simulink model "model_graphicSim"  (R2022a)
settings: Solver=FixedStepAuto  StartTime=0.0  StopTime=inf  RelTol=1e-3
values from neighbouring files (symbols this model uses):
  A = 9    [A_circuit_V2_25000.mat]    (also in A_circuit_V2_3167.mat; A_circuit_V3_30000.mat; A_circuit_V3_60000.mat; Configuration.m)
  d = 699840    [A_circuit_V2_25000.mat]    (also in A_circuit_V2_3167.mat; A_circuit_V3_30000.mat; A_circuit_V3_60000.mat; Configuration.m)
  egoID = 1    [A_circuit_V2_25000.mat]    (also in A_circuit_V2_3167.mat; A_circuit_V3_30000.mat; A_circuit_V3_60000.mat; Configuration.m)
  frontDistCG = 3.7    [A_circuit_V2_25000.mat]    (also in A_circuit_V2_3167.mat; A_circuit_V3_30000.mat; A_circuit_V3_60000.mat; Configuration.m)
  gridvx = [-5 -4.72222222222 -4.44444444444 -4.16666666667 -3.88888888889 -3.61111111111 -3.33333333333 -3.05555555556 -2.77777777778 -2.5 0 0.277777777778 ... (70 elements, 10x7)]    [A_circuit_V2_25000.mat]    (also in A_circuit_V2_3167.mat; A_circuit_V3_30000.mat; A_circuit_V3_60000.mat; circuit_10000_P2.mat)
  gridvy = [-70 -68.4444444444 -66.8888888889 -65.3333333333 -63.7777777778 -62.2222222222 -60.6666666667 -59.1111111111 -57.5555555556 -56 -50 -48.4444444444 ... (70 elements, 10x7)]    [A_circuit_V2_25000.mat]    (also in A_circuit_V2_3167.mat; A_circuit_V3_30000.mat; A_circuit_V3_60000.mat; circuit_10000_P2.mat)
  gridx = [-85 -84.6666666667 -84.3333333333 -84 -83.6666666667 -83.3333333333 -83 -82.6666666667 -82.3333333333 -82 -55 -54.6666666667 ... (70 elements, 10x7)]    [A_circuit_V2_25000.mat]    (also in A_circuit_V2_3167.mat; A_circuit_V3_30000.mat; A_circuit_V3_60000.mat; circuit_10000_P2.mat)
  gridy = [-70 -69.3333333333 -68.6666666667 -68 -67.3333333333 -66.6666666667 -66 -65.3333333333 -64.6666666667 -64 -50 -49.3333333333 ... (70 elements, 10x7)]    [A_circuit_V2_25000.mat]    (also in A_circuit_V2_3167.mat; A_circuit_V3_30000.mat; A_circuit_V3_60000.mat; circuit_10000_P2.mat)
  gridyaw = [-504 -489.6 -475.2 -460.8 -446.4 -432 -417.6 -403.2 -388.8 -374.4 -360 -345.6 ... (70 elements, 10x7)]    [A_circuit_V2_25000.mat]    (also in A_circuit_V2_3167.mat; A_circuit_V3_30000.mat; A_circuit_V3_60000.mat; circuit_10000_P2.mat)
  lb_angSt = -1080    [A_circuit_V2_25000.mat]    (also in A_circuit_V2_3167.mat; A_circuit_V3_30000.mat; A_circuit_V3_60000.mat; Configuration.m = -900)
  lbvx = 0    [A_circuit_V2_25000.mat]    (also in A_circuit_V2_3167.mat; A_circuit_V3_30000.mat; A_circuit_V3_60000.mat; Configuration.m = -2)
  lbvy = -50    [A_circuit_V2_25000.mat]    (also in A_circuit_V2_3167.mat; A_circuit_V3_30000.mat; A_circuit_V3_60000.mat; Configuration.m = -20)
  lbx = -55    [A_circuit_V2_25000.mat]    (also in A_circuit_V2_3167.mat; A_circuit_V3_30000.mat; A_circuit_V3_60000.mat; Configuration.m = 0)
  lby = -50    [A_circuit_V2_25000.mat]    (also in A_circuit_V2_3167.mat; A_circuit_V3_30000.mat; A_circuit_V3_60000.mat; Configuration.m = 2)
  lbyaw = -90    [Configuration.m]    (also in Configuration_circuit.m = -360; Configuration_circuit_V2.m = -360; Configuration_curve.m = -360; Configuration_curve_2.m = -360)
  leftDistCG = 0.9    [A_circuit_V2_25000.mat]    (also in A_circuit_V2_3167.mat; A_circuit_V3_30000.mat; A_circuit_V3_60000.mat; Configuration.m)
  M = 5    [A_circuit_V2_25000.mat]    (also in A_circuit_V2_3167.mat; A_circuit_V3_30000.mat; A_circuit_V3_60000.mat; Configuration.m)
  N = 10    [A_circuit_V2_25000.mat]    (also in A_circuit_V2_3167.mat; A_circuit_V3_30000.mat; A_circuit_V3_60000.mat; Configuration.m)
  passo_steerang = 45    [A_circuit_V2_25000.mat]    (also in A_circuit_V2_3167.mat; A_circuit_V3_30000.mat; A_circuit_V3_60000.mat; Configuration.m = 180)
  passo_v = 0.5    [A_circuit_V2_25000.mat]    (also in A_circuit_V2_3167.mat; A_circuit_V3_30000.mat; A_circuit_V3_60000.mat; Configuration.m)
  retroDistCG = 1    [A_circuit_V2_25000.mat]    (also in A_circuit_V2_3167.mat; A_circuit_V3_30000.mat; A_circuit_V3_60000.mat; Configuration.m)
  safetyDist = 0.5    [A_circuit_V2_25000.mat]    (also in A_circuit_V2_3167.mat; A_circuit_V3_30000.mat; A_circuit_V3_60000.mat; Configuration.m)
  Ts = 0.1    [A_circuit_V2_25000.mat]    (also in A_circuit_V2_3167.mat; A_circuit_V3_30000.mat; A_circuit_V3_60000.mat; Configuration.m)
  ub_angSt = 1080    [A_circuit_V2_25000.mat]    (also in A_circuit_V2_3167.mat; A_circuit_V3_30000.mat; A_circuit_V3_60000.mat; Configuration.m = 900)
  ubvx = 25    [A_circuit_V2_25000.mat]    (also in A_circuit_V2_3167.mat; A_circuit_V3_30000.mat; A_circuit_V3_60000.mat; Configuration.m = 2)
  ubvy = 50    [A_circuit_V2_25000.mat]    (also in A_circuit_V2_3167.mat; A_circuit_V3_30000.mat; A_circuit_V3_60000.mat; Configuration.m = 20)
  ubx = 95    [A_circuit_V2_25000.mat]    (also in A_circuit_V2_3167.mat; A_circuit_V3_30000.mat; A_circuit_V3_60000.mat; Configuration.m = 25)
  uby = 50    [A_circuit_V2_25000.mat]    (also in A_circuit_V2_3167.mat; A_circuit_V3_30000.mat; A_circuit_V3_60000.mat; Configuration.m = 10)
  ubyaw = 90    [Configuration.m]    (also in Configuration_circuit.m = 360; Configuration_circuit_V2.m = 360; Configuration_curve.m = 360; Configuration_curve_2.m = 360)
  w = [0 0 0 0 0 0 0 0 0 0 0 0 ... (699840 elements, 699840x1)]    [A_circuit_V2_25000.mat]    (also in A_circuit_V2_3167.mat; A_circuit_V3_30000.mat; A_circuit_V3_60000.mat; circuit_10000_P2.mat)
  x_0 = 2*rand+19    [Configuration.m]    (also in Configuration_circuit.m = -30; Configuration_circuit_V2.m = 0; Configuration_curve.m = 5; Configuration_curve_2.m = 5)
  y_0 = -(3.5*rand+2)    [Configuration.m]    (also in Configuration_circuit.m = -(-20 - rand*6); Configuration_circuit_V2.m = -(-29.5 - rand*7); Configuration_curve.m = -(1-2.1*rand); Configuration_curve_2.m = -(1-2.1*rand))
undefined symbols (not defined in the file or in its folder): deg, driving, rad, s
libraries: drivingscenarioandsensors x17, simulink_extras x2, sim3dlib x1, sim3dautolib x1, aerolibconvert2 x1, vehdynlibsteering x1, autolibshared x1
(part 1 of 6)
settings Model: Creator=User  LastModifiedBy=User

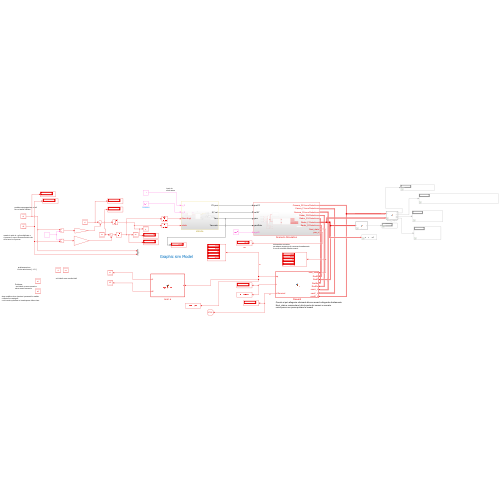
[thumbnail: Simulink's stored preview of the top-level diagram]
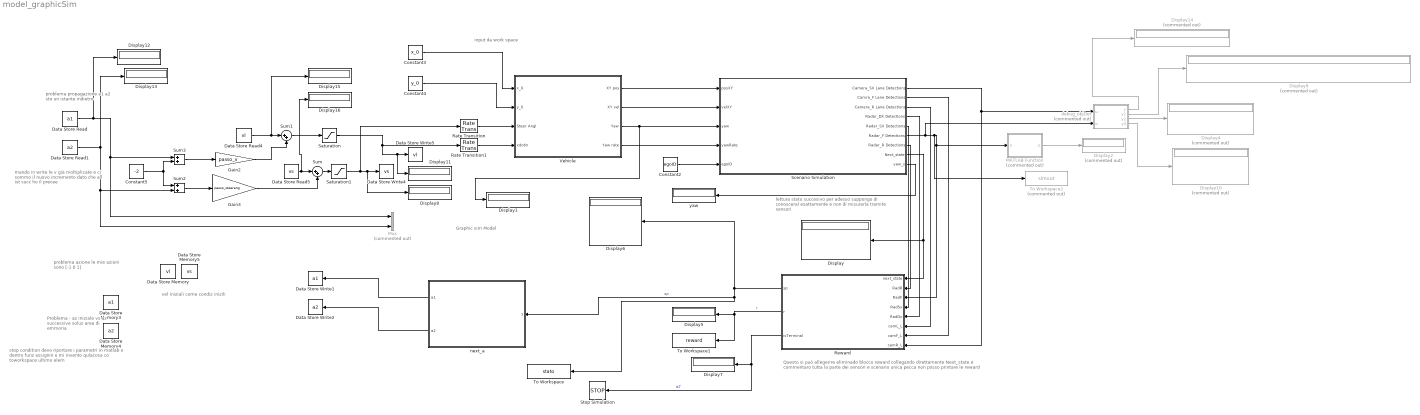
== system model_graphicSim ==
  note: Questo si può allegerire eliminado blocco reward collegando direttamente
      | Next_state e commentaro tutta la parte dei sensori e scenario
      | unica pecca non posso printare le reward
  note: mando in write le v già moltiplicate e
      | ci sommo il nuovo incremento dato che
      | all ist succ ho il precee
  note: problema azione
      | le mie azioni sono [-1 0 1]
  note: vel iniziali come condiz inizili
  note: stop condition devo riportare i parametri in matlab
      | o dentro funz assignin
      | o mi invento qulacosa co toworkspace ultimo elem
  note: Problema
      | - az iniziale vs az successive
      | soluz area di emmoria
  note: problema propagazione a1 a2
      | sto un istante indietro
  note: input da work space
  note: Graphic sim Model
  note: lettura stato succesivo
      | per adesso suppongo di conosceral esattamente
      | e non di misurarla tramite sensori
  Constant2 : Constant  Value=egoID
  Constant3 : Constant  Value=x_0
  Constant4 : Constant  Value=y_0
  Constant5 : Constant  Value=-2
  Data Store Memory : DataStoreMemory  DataStoreName=vl  WriteAfterWriteMsg=warning  ShowAdditionalParam=off
  Data Store Memory3 : DataStoreMemory  DataStoreName=a1  WriteAfterWriteMsg=warning  InitialValue=az_1  VectorParams1D=off  ShowAdditionalParam=off  OutDataTypeStr=double
  Data Store Memory4 : DataStoreMemory  DataStoreName=a2  WriteAfterWriteMsg=warning  InitialValue=az_2  VectorParams1D=off  ShowAdditionalParam=off  OutDataTypeStr=double
  Data Store Memory5 : DataStoreMemory  DataStoreName=vs  WriteAfterWriteMsg=warning  ShowAdditionalParam=off
  Data Store Read : DataStoreRead  DataStoreName=a1  IndexOptions=Index vector (dialog)  Indices=1  OutputSizes=1
  Data Store Read1 : DataStoreRead  DataStoreName=a2  IndexOptions=Index vector (dialog)  Indices=1  OutputSizes=1
  Data Store Read4 : DataStoreRead  DataStoreName=vl  IndexOptions=Index vector (dialog)  Indices=1  OutputSizes=1
  Data Store Read5 : DataStoreRead  DataStoreName=vs  IndexOptions=Index vector (dialog)  Indices=1  OutputSizes=1
  Data Store Write1 : DataStoreWrite  DataStoreName=a1  IndexOptions=Index vector (dialog)  Indices=1  OutputSizes=1
  Data Store Write2 : DataStoreWrite  DataStoreName=a2  IndexOptions=Index vector (dialog)  Indices=1  OutputSizes=1
  Data Store Write4 : DataStoreWrite  DataStoreName=vs  IndexOptions=Index vector (dialog)  Indices=1  OutputSizes=1
  Data Store Write5 : DataStoreWrite  DataStoreName=vl  IndexOptions=Index vector (dialog)  Indices=1  OutputSizes=1
  Display{,1,5..8,11..13,15..16} (11 alike) : Display
  Display{2,4,9..10,14} (5 alike) : Display  Commented=on
  Gain2 : Gain  Gain=passo_v
  Gain3 : Gain  Gain=passo_steerang
  MATLAB Function : MATLAB Function  Commented=on  TreatAsAtomicUnit=on
  Mux : Mux  Commented=on  Inputs=2
  Rate Transition : RateTransition
  Rate Transition1 : RateTransition
  Reward : MATLAB Function  TreatAsAtomicUnit=on
  Saturation : Saturate  UpperLimit=ubvx  LowerLimit=lbvx
  Saturation1 : Saturate  UpperLimit=ub_angSt  LowerLimit=lb_angSt
  Scenario Simulation : Subsystem
  Stop Simulation : Stop
  Sum : Sum  Inputs=|++
  Sum1 : Sum  Inputs=|++
  Sum2 : Sum
  Sum3 : Sum
  To Workspace : ToWorkspace  VariableName=stato  SampleTime=-1
  To Workspace1 : ToWorkspace  VariableName=reward  SampleTime=-1
  To Workspace2 : ToWorkspace  Commented=on  VariableName=simout  SaveFormat=Timeseries  SampleTime=-1
  Vehicle : Subsystem
  debug_objDet : MATLAB Function  Commented=on  TreatAsAtomicUnit=on
  next_a : MATLAB Function  TreatAsAtomicUnit=on
  yaw : Display
  wires:
  Saturation1/1 -> Rate Transition/1, Display8/1, Data Store Write4/1
  Rate Transition/1 -> Vehicle/3(Steer Angl)
  Reward/2(r) -> To Workspace1/1, Display5/1  "r"
  Vehicle/3(Yaw) -> Display1/1, Scenario Simulation/3(yaw)
  Gain2/1 -> Sum1/2
  Sum3/1 -> Gain2/1
  Data Store Read5/1 -> Display16/1, Sum/1
  Data Store Read/1 -> Display12/1, Sum3/1, Mux/1
  Sum1/1 -> Saturation/1
  Sum/1 -> Saturation1/1
  Sum2/1 -> Gain3/1
  Saturation/1 -> Data Store Write5/1, Display11/1, Rate Transition1/1
  Reward/3(isTerminal) -> Stop Simulation/1, Display7/1  "isT"
  Data Store Read1/1 -> Display13/1, Sum2/2, Mux/2
  Constant5/1 -> Sum3/2, Sum2/1
  Gain3/1 -> Sum/2
  Constant3/1 -> Vehicle/1(x_0)
  Data Store Read4/1 -> Display15/1, Sum1/1
  Reward/1(sp) -> Display6/1, To Workspace/1, next_a/1(s)  "sp"
  Vehicle/4(Yaw rate) -> Scenario Simulation/4(yawRate)
  Constant2/1 -> Scenario Simulation/5(egoID)
  Vehicle/2(XY vel) -> Scenario Simulation/2(velXY)
  Rate Transition1/1 -> Vehicle/4(xdotin)
  Vehicle/1(XY pos) -> Scenario Simulation/1(posXY)
  Constant4/1 -> Vehicle/2(y_0)
  next_a/1(a1) -> Data Store Write1/1
  next_a/2(a2) -> Data Store Write2/1
  Scenario Simulation/7(Radar_R Detections) -> Reward/2(RadR)
  Scenario Simulation/5(" Radar_SX Detections") -> Reward/4(RadSx)
  Scenario Simulation/4(Radar_DX Detections) -> Reward/5(RadDx)
  Scenario Simulation/3(Camera_R Lane Detections) -> Reward/6(camL_L)
  Scenario Simulation/2(" Camra_F Lane Detections") -> Reward/7(camF_L)
  Scenario Simulation/1(Camera_SX Lane Detections) -> debug_objDet/1(u), Reward/8(camR_L)
  Scenario Simulation/8(Next_state) -> Display/1, Reward/1(next_state)
  Scenario Simulation/9(yaw_s) -> yaw/1
  Scenario Simulation/6(Radar_F Detections) -> debug_objDet/2(o), MATLAB Function/1(u), Reward/3(RadF), To Workspace2/1
  MATLAB Function/1(y) -> Display2/1
  debug_objDet/4(y3) -> Display10/1
  debug_objDet/1(y) -> Display14/1
  debug_objDet/3(y2) -> Display4/1
  debug_objDet/2(y1) -> Display9/1

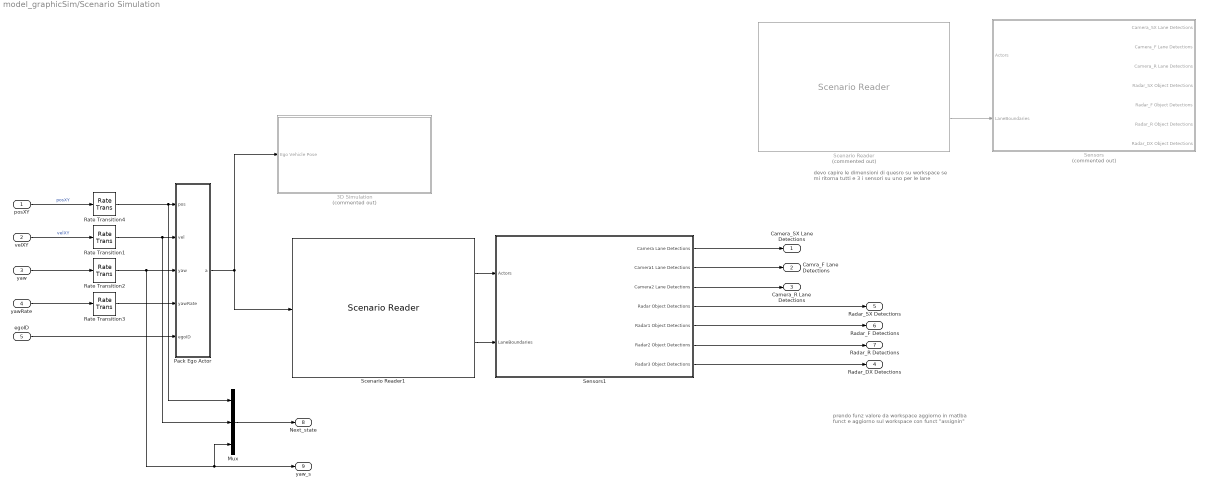
== system model_graphicSim/Scenario Simulation ==
  note: devo capire le dimensioni di quesro su workspace
      | se mi ritorna tutti e 3 i sensori su uno per le lane
  note: prendo funz valore da workspace
      | aggiorno in matlba funct e aggiorno sul workspace
      | con funct "assignin"
  posXY : Inport
  velXY : Inport  Port=2
  yaw : Inport  Port=3
  yawRate : Inport  Port=4
  egoID : Inport  Port=5
  3D Simulation : Subsystem  Commented=on
  Mux : Mux  Inputs=3
  Pack Ego Actor : MATLAB Function  TreatAsAtomicUnit=on
  Rate Transition{1..4} (4 alike) : RateTransition  OutPortSampleTime=Ts
  Scenario Reader : drivingscenarioandsensors/Scenario Reader  Commented=on  ScenarioSource=From file  ScenarioFileName=C:\Users\User\OneDrive\Desktop\Thesis_Project\project\parking_Scenario_withRadar.mat  ScenarioVariableName=scenario  OutputCoordinateSystem=Vehicle coordinates  EgoVehicleSource=Input port  EgoVehicleActorID=1  OrientVehiclesOnRoad=off  OutputEgoVehiclePose=off  OutputEgoVehicleState=off  SampleTime=Ts  LaneBoundaryOutput=Ego vehicle lane boundaries  LaneBoundaryDistance=linspace(-150, 150, 101)  LaneBoundaryLocation=Center of lane markings  BusNameSource=Auto  BusName=BusActors  BusNumActorsSource=Scenario  BusNumActors=100  BusName2Source=Auto  BusName2=BusLaneBoundaries  BusNumLaneBoundariesSource=Scenario  BusNumLaneBoundaries=10  BusName3Source=Auto  BusName3=BusEgoActor  BusName4Source=Auto  BusName4=BusEgoState  ShowCoordinateLabels=on  SimulateUsing=Interpreted execution
  Scenario Reader1 : drivingscenarioandsensors/Scenario Reader  ScenarioSource=From file  ScenarioFileName=C:\Users\User\OneDrive\Desktop\ThesisProject\project\parking_Scenario_withRadar.mat  ScenarioVariableName=scenario  OutputCoordinateSystem=Vehicle coordinates  EgoVehicleSource=Input port  EgoVehicleActorID=1  OrientVehiclesOnRoad=off  OutputEgoVehiclePose=off  OutputEgoVehicleState=off  SampleTime=0.1  LaneBoundaryOutput=Ego vehicle lane boundaries  LaneBoundaryDistance=linspace(-150, 150, 101)  LaneBoundaryLocation=Center of lane markings  BusNameSource=Auto  BusName=BusActors  BusNumActorsSource=Scenario  BusNumActors=100  BusName2Source=Auto  BusName2=BusLaneBoundaries  BusNumLaneBoundariesSource=Scenario  BusNumLaneBoundaries=10  BusName3Source=Auto  BusName3=BusEgoActor  BusName4Source=Auto  BusName4=BusEgoState  ShowCoordinateLabels=on  SimulateUsing=Interpreted execution
  Sensors : Subsystem  Commented=on
  Sensors1 : Subsystem
  Camera_SX Lane Detections : Outport
  " Camra_F Lane Detections" : Outport  Port=2
  Camera_R Lane Detections : Outport  Port=3
  Radar_DX Detections : Outport  Port=4
  " Radar_SX Detections" : Outport  Port=5
  Radar_F Detections : Outport  Port=6
  Radar_R Detections : Outport  Port=7
  Next_state : Outport  Port=8
  yaw_s : Outport  Port=9
  wires:
  Pack Ego Actor/1(a) -> Scenario Reader1/1, 3D Simulation/1(Ego Vehicle Pose)
  Sensors1/5(Radar1 Object Detections) -> Radar_F Detections/1
  yawRate/1 -> Rate Transition3/1
  Rate Transition1/1 -> Mux/2, Pack Ego Actor/2(vel)
  Rate Transition4/1 -> Mux/1, Pack Ego Actor/1(pos)
  Rate Transition3/1 -> Pack Ego Actor/4(yawRate)
  Rate Transition2/1 -> Mux/3, yaw_s/1, Pack Ego Actor/3(yaw)
  egoID/1 -> Pack Ego Actor/5(egoID)
  velXY/1 -> Rate Transition1/1  "velXY"
  posXY/1 -> Rate Transition4/1  "posXY"
  yaw/1 -> Rate Transition2/1
  Sensors1/1(Camera Lane Detections) -> Camera_SX Lane Detections/1
  Sensors1/2(Camera1 Lane Detections) -> " Camra_F Lane Detections"/1
  Sensors1/3(Camera2 Lane Detections) -> Camera_R Lane Detections/1
  Sensors1/4(Radar Object Detections) -> " Radar_SX Detections"/1
  Sensors1/6(Radar2 Object Detections) -> Radar_R Detections/1
  Sensors1/7(Radar3 Object Detections) -> Radar_DX Detections/1
  Mux/1 -> Next_state/1
  Scenario Reader/2 -> Sensors/2(LaneBoundaries)
  Scenario Reader1/1 -> Sensors1/1(Actors)
  Scenario Reader1/2 -> Sensors1/2(LaneBoundaries)

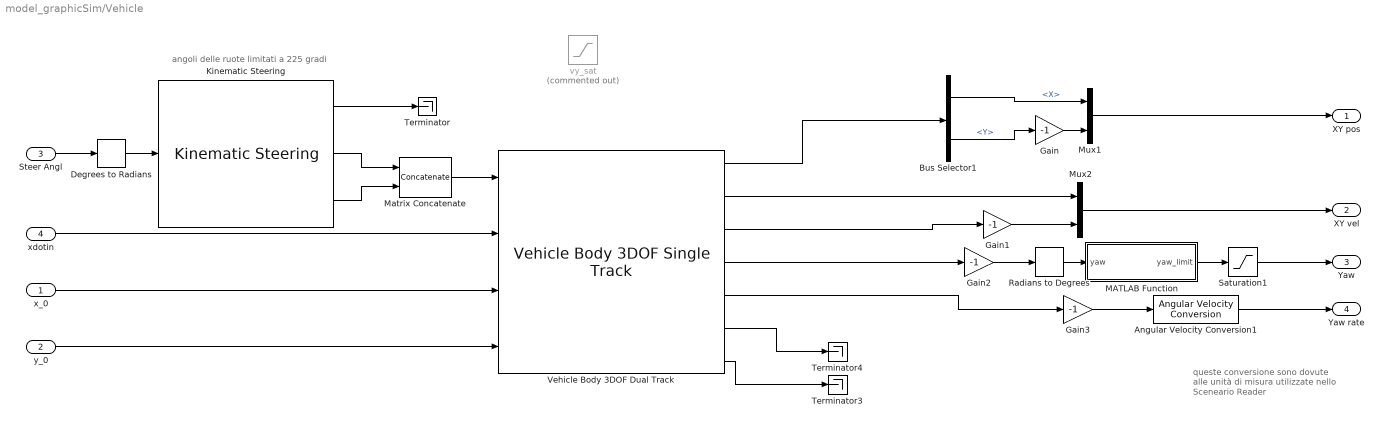
== system model_graphicSim/Vehicle ==
  note: angoli delle ruote limitati a 225 gradi
  note: queste conversione sono dovute
      | alle unità di misura utilizzate nello
      | Sceneario Reader
  x_0 : Inport
  y_0 : Inport  Port=2
  Steer Angl : Inport  Port=3
  xdotin : Inport  Port=4
  Angular Velocity Conversion1 : aerolibconvert2/Angular Velocity Conversion  IU=rad/s  OU=deg/s
  Bus Selector1 : BusSelector  OutputSignals=InertFrm.Cg.Disp.X,InertFrm.Cg.Disp.Y
  Degrees to Radians : simulink_extras/Transformations/Degrees to Radians
  Gain{,1..3} (4 alike) : Gain  Gain=-1
  Kinematic Steering : vehdynlibsteering/Kinematic Steering  StrgType=Ackerman  StrgRatioType=Constant  Loc=Front  NrmlFctr=0.01  TrckWdth=1  WhlBase=1.524  Db=0  StrgRng=5*pi  StrgAngBpts="[-6.2832   -5.0265   -3.7699   -2.5133   -1.2566         0    1.2566    2.5133    3.7699    5.0265    6.2832]"  StrgRatioTbl=|  StrgRatio=100  PctAckIn=off  PctAck=100  PctAckTbl=ones(1,11)*100  StrgArmLngth=0.1  RckCsLngth=0.5  TieRodLngth=0.248  D=0.2  PnnRadius=0.00085818  PnnRadiusTbl="[0.0055    0.0055    0.0056    0.0057    0.0058    0.0057    0.0057    0.0057    0.0056    0.0055    0.0055]"  RodLngth=0.1  ParaArmLngth=0.9  aMode=2
      | [13.5000   13.3750   13.2500   13.1250   13.0000   13.0000   13.0000   13.1250   13.2500   13.3750   13.5000
      | ]
  MATLAB Function : MATLAB Function  TreatAsAtomicUnit=on
  Matrix Concatenate : Concatenate  ConcatenateDimension=2
  Mux1 : Mux  Inputs=2
  Mux2 : Mux  Inputs=2
  Radians to Degrees : simulink_extras/Transformations/Radians to Degrees
  Saturation1 : Saturate  UpperLimit=360  LowerLimit=-360
  Terminator : Terminator
  Terminator3 : Terminator
  Terminator4 : Terminator
  Vehicle Body 3DOF Dual Track : autolibshared/Vehicle Body 3DOF Single Track  trackMode=Dual  inputMode=External longitudinal velocity  frontSteerMode=on  rearSteerMode=off  windMode=off  muMode=off  extFMode=off  extMMode=off  htchFMode=off  htchMMode=off  extXo=on  extpsio=off  extxdoto=off  extro=off  extYo=on  extTamb=off  extydoto=off  aMode=2  NF=2  NR=2  m=2000  a=1.4  b=1.6  h=0.35  dh=1  hh=0.2  X_o=0  xdot_o=0  CalphaMode=off  sigmaMode=on  d=0  hl=0  w=[1.4,1.4]  Cy_f=12e3  Cy_r=11e3  sigma_f=.1  sigma_r=.1  alpha_f_brk=[-.1 .1]  Cy_f_data=[-9e3 9e3]  alpha_r_brk=[-.1 .1]  Cy_r_data=[-9e3 9e3]  Y_o=0  ydot_o=0  Izz=4000  psi_o=0  r_o=0  Af=2  Cd=.3  Cl=.1  Cpm=.1  beta_w=[0 0.01:0.01:0.3]  Cs=[0:0.03:0.9]  Cym=[0 1e-6:0.01:0.3]  Pabs=101325  Tair=273  g=9.81  mu=1  xdot_tol=.01  Fznom=5000  Fxtire_sat=7e4  Fytire_sat=7e4  longOff=0  latOff=0  vertOff=0  wrapAng=off
      settings: SourceProductBaseCode=PW,DR,MT,VE
  vy_sat : Saturate  Commented=on  UpperLimit=ubvy  LowerLimit=lbvy
  XY pos : Outport
  XY vel : Outport  Port=2
  Yaw : Outport  Port=3
  Yaw rate : Outport  Port=4
  wires:
  Bus Selector1/2 -> Gain/1  "<Y>"
  Kinematic Steering/3 -> Matrix Concatenate/2
  Matrix Concatenate/1 -> Vehicle Body 3DOF Dual Track/1
  Vehicle Body 3DOF Dual Track/6 -> Terminator4/1
  Mux1/1 -> XY pos/1
  Bus Selector1/1 -> Mux1/1  "<X>"
  Kinematic Steering/1 -> Terminator/1
  Degrees to Radians/1 -> Kinematic Steering/1
  Vehicle Body 3DOF Dual Track/7 -> Terminator3/1
  Kinematic Steering/2 -> Matrix Concatenate/1
  Mux2/1 -> XY vel/1
  Steer Angl/1 -> Degrees to Radians/1
  xdotin/1 -> Vehicle Body 3DOF Dual Track/2
  Radians to Degrees/1 -> MATLAB Function/1(yaw)
  Gain3/1 -> Angular Velocity Conversion1/1
  x_0/1 -> Vehicle Body 3DOF Dual Track/3
  y_0/1 -> Vehicle Body 3DOF Dual Track/4
  Vehicle Body 3DOF Dual Track/3 -> Gain1/1
  MATLAB Function/1(yaw_limit) -> Saturation1/1
  Saturation1/1 -> Yaw/1
  Vehicle Body 3DOF Dual Track/2 -> Mux2/1
  Vehicle Body 3DOF Dual Track/1 -> Bus Selector1/1
  Gain/1 -> Mux1/2
  Gain1/1 -> Mux2/2
  Gain2/1 -> Radians to Degrees/1
  Vehicle Body 3DOF Dual Track/5 -> Gain3/1
  Vehicle Body 3DOF Dual Track/4 -> Gain2/1
  Angular Velocity Conversion1/1 -> Yaw rate/1

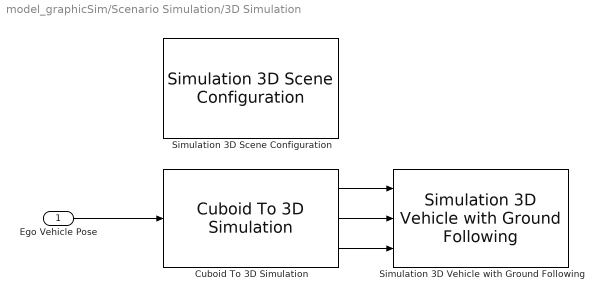
== system model_graphicSim/Scenario Simulation/3D Simulation ==
  Ego Vehicle Pose : Inport
  Cuboid To 3D Simulation : drivingscenarioandsensors/Cuboid To 3D Simulation  SpecifyActorID=on  ActorIDToConvert=1  SimulateUsing=Interpreted execution
      settings: SourceProductBaseCode=DR
  Simulation 3D Scene Configuration : sim3dlib/Simulation 3D Scene Configuration  Priority=0  ProjectFormat=Default Scenes  SceneDesc=Straight road  ProjectName=C:\Program Files\MATLAB\R2022a\toolbox\shared\sim3d_projects\automotive_project\UE4\WindowsNoEditor\VehicleSimulation.exe  ScenePath=/Game/Maps/HwStrght  vehTagList={'Scene Origin';'SimulinkVehicle1'}  vehTag=SimulinkVehicle1  OpVisEn=off  Ts=1/60  EnableWindow=on  EnableRemoteAccess=off  EnableWeather=off  SunAltitude=40.0  SunAzimuth=90  clouds=10  wind=1  fog=0  rain=0  sensorTag=MainCamera1  sensorId=1  sensorName=MainCamera1  mountLoc=Origin  offsetFlag=off  tmountOffset=[0, 0, 0]  rmountOffset=[0, 0, 0]  HorizontalResolution=1280  VerticalResolution=720  HorizontalFOV=60  mountPoint=[0 0 0]  mountOrientation=[0 0 0]  aMode=3  ID=1
      settings: SourceProductBaseCode=VE,AE,DR,UV,VE
  Simulation 3D Vehicle with Ground Following : sim3dautolib/Simulation 3D Vehicle with Ground Following  Priority=-1  PassVehMesh=Muscle car  MeshPath=/MathWorksSimulation/Vehicles/Muscle/Meshes/SK_MuscleCar.SK_MuscleCar  TrackWidth=1.9  WheelBase=3  WheelRadius=0.35  VehColor=Red  InitialPos=[0, 0, 0]  InitialRot=[0, 0, 0]  ActorName=SimulinkVehicle1  SampleTime=-1  ActorType=SimulinkVehicle  ID=1  aMode=3  ActorTag=SimulinkVehicle1  CoordinateScheme=ISO  VehLightsControl=off  HeadlightColor=[ 1, 1, 1 ]  HighBeamIntensity=100000  LowBeamIntensity=60000  HighBeamConeAngle=70  LowBeamConeAngle=70  LeftHeadlightOrientation=[ 0, 0 ]  RightHeadlightOrientation=[ 0, 0 ]  BrakelightIntensity=500  ReverselightIntensity=500  SignallightIntensity=500  SignallightPeriod=1  SignalPulseWidth=50  TransformOutportEnabled=off
      settings: SourceProductBaseCode=VE,AE,DR,UV,VE
  wires:
  Cuboid To 3D Simulation/3 -> Simulation 3D Vehicle with Ground Following/3
  Cuboid To 3D Simulation/2 -> Simulation 3D Vehicle with Ground Following/2
  Cuboid To 3D Simulation/1 -> Simulation 3D Vehicle with Ground Following/1
  Ego Vehicle Pose/1 -> Cuboid To 3D Simulation/1
